simulink model "zajecia4simulink"  (R2022b)
settings: Solver=VariableStepAuto  StartTime=0.0  StopTime=t_simulation  RelTol=1e-3
values from neighbouring files (symbols this model uses):
  Cvp = cp * rop * Vp    (= 46080)    [zajecia4matlab.m]
  Cvw = cp * rop * Vw    (= 76800)    [zajecia4matlab.m]
  dgq = 0.1 * qgN    (= 1000)    [zajecia4matlab.m]
  dTzew = 0    [zajecia4matlab.m]
  Kcp = (qgN/(TwewN * (1 + a) - TzewN - a * TpN))  * (a * (TwewN - TpN))/(TpN -  TzewN)    (= 19.6078431373)    [zajecia4matlab.m]
  Kcw = qgN/(TwewN * (1 + a) - TzewN - a * TpN)    (= 235.294117647)    [zajecia4matlab.m]
  Kcwp = a*qgN/(TwewN*(1+a) -TzewN - a*TpN)    (= 58.8235294118)    [zajecia4matlab.m]
  LTp11 = K0Tp    (= 0.003)    [zajecia4matlab.m]
  LTp11DP = K0TpDP    (= 0.003)    [zajecia4matlab.m]
  LTwew11 = K0Twew    (= 0.004)    [zajecia4matlab.m]
  LTwew11DP = K0TwewDP    (= 0.004)    [zajecia4matlab.m]
  MTp11 = [TTp 1]    [zajecia4matlab.m]
  MTp11DP = [TTpDP 1]    [zajecia4matlab.m]
  MTwew11 = [TTwew 1]    [zajecia4matlab.m]
  MTwew11DP = [TTwewDP 1]    [zajecia4matlab.m]
  qg0 = qgN    (= 10000)    [zajecia4matlab.m]
  t0 = 500    [zajecia4matlab.m]
  Tp0 = (Kcp*Tzew0 + Kcwp * Twew0)/(Kcwp + Kcp)    (= 10)    [zajecia4matlab.m]
  Twew0 = ((qg0*(Kcp + Kcwp))/(Kcwp*Kcw + Kcp * Kcw + Kcp * Kcwp)) + Tzew0    (= 20)    [zajecia4matlab.m]
  Tzew0 = TzewN    (= -20)    [zajecia4matlab.m]
settings Model: Creator=huber  LastModifiedBy=huber
settings DataIOCC: ReturnWorkspaceOutputs=off

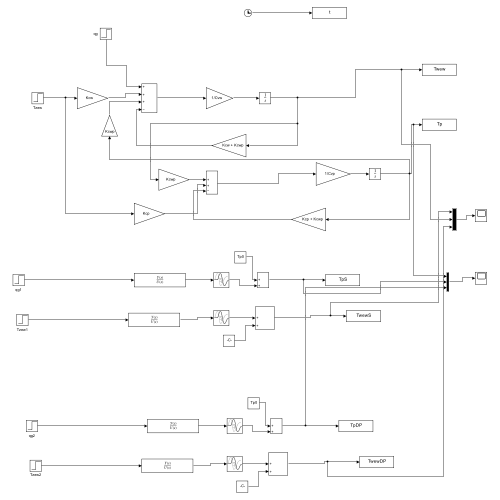
[thumbnail: Simulink's stored preview of the top-level diagram]
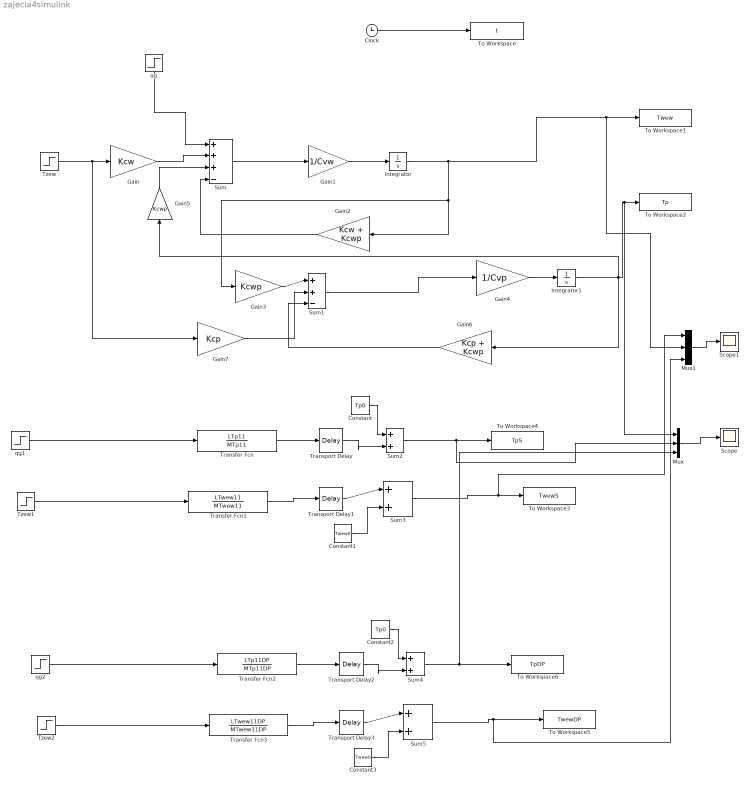
== system zajecia4simulink ==
  Clock : Clock
  Constant : Constant  Value=Tp0
  Constant1 : Constant  Value=Twew0
  Constant2 : Constant  Value=Tp0
  Constant3 : Constant  Value=Twew0
  Gain : Gain  Gain=Kcw
  Gain1 : Gain  Gain=1/Cvw
  Gain2 : Gain  Gain=Kcw + Kcwp
  Gain3 : Gain  Gain=Kcwp
  Gain4 : Gain  Gain=1/Cvp
  Gain5 : Gain  Gain=Kcwp
  Gain6 : Gain  Gain=Kcp + Kcwp
  Gain7 : Gain  Gain=Kcp
  Integrator : Integrator  InitialCondition=Twew0
  Integrator1 : Integrator  InitialCondition=Tp0
  Mux : Mux  Inputs=3
  Mux1 : Mux  Inputs=3
  Scope : Scope
  Scope1 : Scope
  Sum : Sum  Inputs=+++-
  Sum1 : Sum  Inputs=|++-
  Sum{2..5} (4 alike) : Sum  Inputs=|++
  To Workspace : ToWorkspace  VariableName=t  SampleTime=-1
  To Workspace1 : ToWorkspace  VariableName=Twew  SampleTime=-1
  To Workspace2 : ToWorkspace  VariableName=Tp  SampleTime=-1
  To Workspace3 : ToWorkspace  VariableName=TwewS  SampleTime=-1
  To Workspace4 : ToWorkspace  VariableName=TpS  SampleTime=-1
  To Workspace5 : ToWorkspace  VariableName=TwewDP  SampleTime=-1
  To Workspace6 : ToWorkspace  VariableName=TpDP  SampleTime=-1
  Transfer Fcn : TransferFcn  Numerator=LTp11  Denominator=MTp11
  Transfer Fcn1 : TransferFcn  Numerator=LTwew11  Denominator=MTwew11
  Transfer Fcn2 : TransferFcn  Numerator=LTp11DP  Denominator=MTp11DP
  Transfer Fcn3 : TransferFcn  Numerator=LTwew11DP  Denominator=MTwew11DP
  Transport Delay{,1..3} (4 alike) : TransportDelay  DelayTime=0
  Tzew : Step  Time=t0  Before=Tzew0  After=Tzew0 + dTzew  SampleTime=0
  Tzew1 : Step  Time=t0  After=dgq  SampleTime=0
  Tzew2 : Step  Time=t0  After=dgq  SampleTime=0
  qg : Step  Time=t0  Before=qg0  After=qg0 + dgq  SampleTime=0
  qg1 : Step  Time=t0  After=dgq  SampleTime=0
  qg2 : Step  Time=t0  After=dgq  SampleTime=0
  wires:
  Clock/1 -> To Workspace/1
  Tzew/1 -> Gain7/1, Gain/1
  Gain/1 -> Sum/2
  Sum/1 -> Gain1/1
  Gain1/1 -> Integrator/1
  Gain2/1 -> Sum/4
  qg/1 -> Sum/1
  Integrator/1 -> Gain3/1, Gain2/1, Mux1/2, To Workspace1/1
  Gain3/1 -> Sum1/1
  Sum1/1 -> Gain4/1
  Gain4/1 -> Integrator1/1
  Gain6/1 -> Sum1/3
  Gain5/1 -> Sum/3
  Gain7/1 -> Sum1/2
  qg1/1 -> Transfer Fcn/1
  Transfer Fcn/1 -> Transport Delay/1
  Constant/1 -> Sum2/1
  Transport Delay/1 -> Sum2/2
  Tzew1/1 -> Transfer Fcn1/1
  Transport Delay1/1 -> Sum3/1
  Transfer Fcn1/1 -> Transport Delay1/1
  Constant1/1 -> Sum3/2
  Sum2/1 -> Mux/2, To Workspace4/1
  Sum3/1 -> Mux1/1, To Workspace3/1
  Integrator1/1 -> Gain5/1, Gain6/1, Mux/1, To Workspace2/1
  Mux1/1 -> Scope1/1
  Mux/1 -> Scope/1
  Transport Delay2/1 -> Sum4/2
  Constant2/1 -> Sum4/1
  Sum4/1 -> Mux/3, To Workspace6/1
  Transfer Fcn3/1 -> Transport Delay3/1
  Transfer Fcn2/1 -> Transport Delay2/1
  Constant3/1 -> Sum5/2
  qg2/1 -> Transfer Fcn2/1
  Tzew2/1 -> Transfer Fcn3/1
  Transport Delay3/1 -> Sum5/1
  Sum5/1 -> Mux1/3, To Workspace5/1
